simulink model "effect_of_controller_on_signal_step_signal"  (R2019a)
settings: Solver=VariableStepAuto  StartTime=0.0  StopTime=15  RelTol=1e-3
libraries: dspsrcs4 x1, simulink x1
settings Model: Creator=raxit  LastModifiedBy=raxit

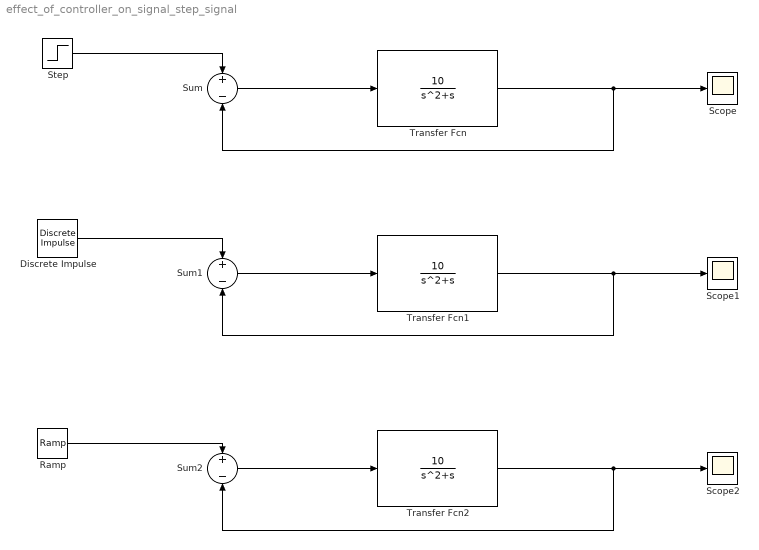
== system effect_of_controller_on_signal_step_signal ==
  Discrete Impulse : dspsrcs4/Discrete  Impulse  Delay=0  SampleTime=1  FrameSample=1  OutputFrames=off  dataType=double  isSigned=on  wordLen=16  udDataType=sfix(16)  fracBitsMode=Best precision  numFracBits=15  OutDataTypeStr=double  LastOutDataTypeStr=double
  Ramp : simulink/Sources/Ramp  slope=1  start=0  InitialOutput=0
  Scope : Scope
  Scope1 : Scope
  Scope2 : Scope
  Step : Step  SampleTime=0
  Sum : Sum  Inputs=+-
  Sum1 : Sum  Inputs=+-
  Sum2 : Sum  Inputs=+-
  Transfer Fcn : TransferFcn  Numerator=[10]  Denominator=[1 1 0]
  Transfer Fcn1 : TransferFcn  Numerator=[10]  Denominator=[1 1 0]
  Transfer Fcn2 : TransferFcn  Numerator=[10]  Denominator=[1 1 0]
  wires:
  Sum/1 -> Transfer Fcn/1
  Transfer Fcn/1 -> Sum/2, Scope/1
  Step/1 -> Sum/1
  Discrete Impulse/1 -> Sum1/1
  Transfer Fcn1/1 -> Sum1/2, Scope1/1
  Sum1/1 -> Transfer Fcn1/1
  Ramp/1 -> Sum2/1
  Transfer Fcn2/1 -> Sum2/2, Scope2/1
  Sum2/1 -> Transfer Fcn2/1
